simulink library "fit6DoF_ul"  (R2018b)
settings: Solver=VariableStepAuto  StartTime=0.0  StopTime=10.0  RelTol=1e-3
settings Model: Creator=M.Cobb  LastModifiedBy=M.Cobb

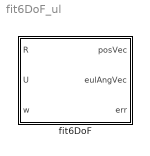
== system fit6DoF_ul ==
  fit6DoF : Subsystem  mask{D=0, initPosVec=[0 0 50], initEulAng=[0 0 0]*pi/180, HInvInit=eye(6), maxIBFGS=20, posTolBFGS=0.05, angTolBFGS=0.05*pi/180, dxPos=0.0001*[1 1 1], dxEul=0.01*[1 1 1]*pi/180, stepSize=1e-4, maxIBP=100, maxIGS=1000, posTolGS=0.05, angTolGS=0.05*pi/180}
      mask prompts: D "Dot position vector matrix"; initPosVec "Initial position vector guess [cm]"; initEulAng "Initial Euler angle vector guess, (roll, pitch, yaw) [rad]"; HInvInit "Initial guess inverse Hessian"; maxIBFGS "Max num of iterations"; posTolBFGS "Position tolerance [cm]"; angTolBFGS "Angular tolerance [rad]"; dxPos "Position perturbation size [cm]"; dxEul "Euler angle perturbation size [rad]"; stepSize "Initial step size"; maxIBP "Max num of iterations"; maxIGS "Max num of iterations"; posTolGS "Position tolerance [cm]"; angTolGS "Angular tolerance [cm]"
      mask help:
      | Block to resolve position of the CM relative to the ground origin (in cm) and euler angles (roll pitch yaw, in rad) using the BFGS-based numerical minimization technique.
      |
      | See help for more.
      mask Help:
      | In this documentation, N is the number of dots being tracked (8 at the time of writing).
      | 
      | Input Signals Obtained from Ray Tracing:
      | R: 3 by N matrix of ray position vectors.  Each column is a vector from the ground origin to the point where the ray exits the glass and enters the water.
      | U: 3 by N matrix of ray unit vectors.  Each column is a unit vector that describes the direction of the ray.
      | w: N by 1 vector of weights used in the performance index.  w_i is the weight applied to the result of the i-th ray trace.  Can be used to ignore bad ray tracing or image processing results in the numerical solution.
      mask DialogControl D Tooltip: 3 by N matrix, where N is the number of dots being tracked.  Matrix is columns are CG to dot pos vecs in body frame.
      mask DialogControl ParameterGroupVar Prompt: BFGS Parameters
      mask DialogControl initPosVec Tooltip: Guess on first time step.  Algorithm reverts to this in the event of an error.
      mask DialogControl initEulAng Tooltip: Guess on first time step.  Algorithm reverts to this in the event of an error.
      mask DialogControl posTolBFGS Tooltip: BFGS step size must be smaller than ball of this radius
      mask DialogControl angTolBFGS Tooltip: BFGS step size must be smaller than ball of this radius
      mask DialogControl Container3 Prompt: Numerical gradient
      mask DialogControl Container4 Prompt: Bounding phase parameters
      mask DialogControl Container6 Prompt: Golden section parameters

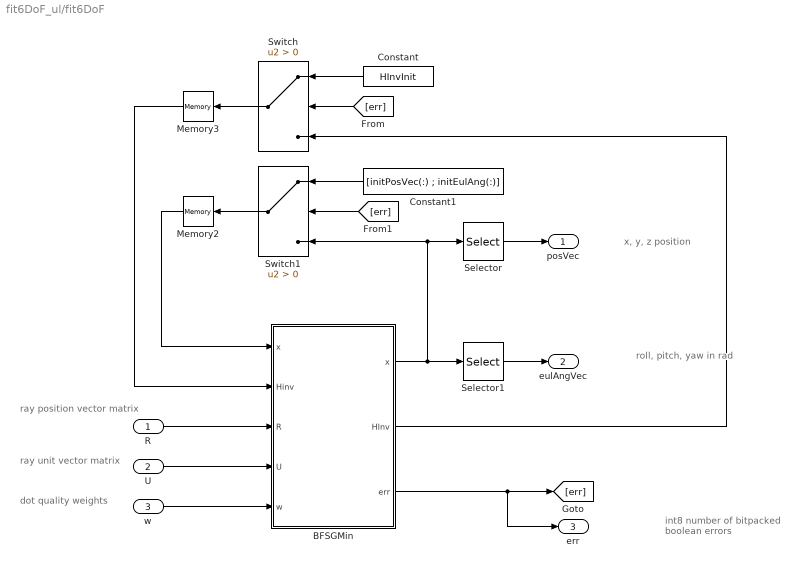
== system fit6DoF_ul/fit6DoF ==
  note: ray position
      | vector matrix
  note: int8 number of bitpacked
      | boolean errors
  note: x, y, z position
  note: roll, pitch, yaw
      | in rad
  note: ray unit
      | vector matrix
  note: dot quality
      | weights
  R : Inport
  U : Inport  Port=2
  w : Inport  Port=3
  BFSGMin : MATLAB Function  TreatAsAtomicUnit=on
  Constant : Constant  Value=HInvInit
  Constant1 : Constant  Value=[initPosVec(:) ; initEulAng(:)]
  Memory2 : Memory  InitialCondition=[initPosVec(:) ; initEulAng(:)]  InheritSampleTime=on
  Memory3 : Memory  InitialCondition=HInvInit  InheritSampleTime=on
  Selector : Selector  InputPortWidth=6  IndexOptions=Index vector (dialog)  Indices=1:3  OutputSizes=1
  Selector1 : Selector  InputPortWidth=6  IndexOptions=Index vector (dialog)  Indices=4:6  OutputSizes=1
  Switch : Switch  Criteria=u2 > Threshold
  Switch1 : Switch  Criteria=u2 > Threshold
  posVec : Outport
  eulAngVec : Outport  Port=2
  err : Outport  Port=3
  wires:
  R/1 -> BFSGMin/3(R)
  U/1 -> BFSGMin/4(U)
  w/1 -> BFSGMin/5(w)
  BFSGMin/3(err) -> err/1, [err]
  Selector/1 -> posVec/1
  Selector1/1 -> eulAngVec/1
  BFSGMin/2(HInv) -> Switch/3
  BFSGMin/1(x) -> Switch1/3, Selector/1, Selector1/1
  [err] -> Switch/2
  Constant/1 -> Switch/1
  [err] -> Switch1/2
  Constant1/1 -> Switch1/1
  Switch1/1 -> Memory2/1
  Switch/1 -> Memory3/1
  Memory2/1 -> BFSGMin/1("x ")
  Memory3/1 -> BFSGMin/2(Hinv)

== matlab function fit6DoF_ul/fit6DoF/BFSGMin ==
  data: x input size=[6 1]; x output; Hinv input size=[6 6]; R input; U input; w input; HInv output; err output int8 size=1; dxPos parameter; dxEul parameter; stepSize parameter; maxIBFGS parameter; maxIGS parameter; maxIBP parameter; posTolBFGS parameter; posTolGS parameter; angTolBFGS parameter; angTolGS parameter; D parameter
function [x,HInv,err] = fcn(x,Hinv,R,U,w,...
    dxPos, dxEul,stepSize,...
    maxIBFGS, maxIGS, maxIBP,...
    posTolBFGS, posTolGS,...
    angTolBFGS, angTolGS, D)

%#codegen
[x,HInv,err] = BFGS(x(:),Hinv,R,D,U,w,...
    [dxPos(:) ; dxEul(:)],stepSize,...
    maxIBFGS,maxIGS,maxIBP,...
    posTolBFGS,posTolGS,...
    angTolBFGS,angTolGS);
